simulink model "TEST_simulink"  (R2022b)
settings: Solver=VariableStepAuto  StartTime=0.0  StopTime=10.0  RelTol=1e-3
undefined symbols (not defined in the file): c0, c1, GFl_Final_vlaue, GFl_Initial_value, GFl_P_primary, GFl_Q_set, GFl_Sample_time, GFl_Step_time, GFm_Final_vlaue, GFm_Initial_value, GFm_P_primary, GFm_Q_set, GFm_Sample_time, GFm_Step_time, GFm_V_set_phph, GFmAIC_f_set, GFmAIC_Final_vlaue, GFmAIC_Initial_value, GFmAIC_P_primary, GFmAIC_P_set, GFmAIC_Q_set, GFmAIC_Sample_time, GFmAIC_Step_time, l0, l1, r0, r1, SG_f_set, SG_Final_vlaue, SG_Initial_value, SG_P_primary, SG_Q_set, SG_Sample_time, SG_Step_time, SG_V_set_phph, sigbuilder_block, V1_L1, V1_Ph_Ph, V1_R1, V2_L1, V2_Ph_Ph, V2_R1
libraries: Model_DG_Grid_Forming_Converter x30, Model_DG_Grid_Following_Converter x15, simulink x15, Model_DG_Synchronous_Generator x15, spsThreePhaseVIMeasurementLib x14, spsThreePhasePISectionLineLib x14, spsThreePhaseBreakerLib x6, spsThreePhaseFaultLib x3, spsThreePhaseParallelRLCLoadLib x2, spsThreePhaseTransformerTwoWindingsLib x2, spspowerguiLib x1
(part 4 of 6)

== system TEST_simulink/DER 2/Grid Forming Conventer ==
  Bus Selector : BusSelector  OutputSignals=controller.measurements.P_grid,controller.measurements.Q_grid,controller.inner_control.f,physical.V_dc,physical.V_grid_abc
  Constant : Constant  Value=GFm_P_primary
  Constant10 : Constant  Value=GFm_Q_set
  Constant4 : Constant  Value=GFmAIC_f_set
  Constant6 : Constant  Value=GFm_V_set_phph
  Grid_Forming_Converter1 : Model_DG_Grid_Forming_Converter/Grid_Forming_Converter  S_n=2e6  V_n_phph=690  f_n=50  send_messages=on  T_s_ctrl=1e-4  T_s_PWM_meas=1e-4  T_s_SPS=1e-4  datatype='double'  swModeling=Average Model  f_sw=5e3  L_filter_conv_pu=[ 0.001 0.05097 ]  C_filter_pu=[ 0.06875 0.04569 ]  L_filter_grid_pu=[ 0.01 0.04 ]  C_dc_pu=0.75  withTransformer=Grid coupling using transformer  V_n_grid_phph=20e3  RL_Trafo_Conv=[ 0.005 0.02 ]  RL_Trafo_Grid=[ 0.005 0.02 ]  Rm=500  Lm=500  meas_lowpass=on  meas_f_cutoff_lowpass=2500  meas_f_cutoff_posseq=20  prot_variant=tDMSquared warnings only  v_dc_max=1.2  v_ac_max=1.4  t_ac_max=0.1  v_ac_maxmax=1.25  t_ac_maxmax=0.1  v_ac_min=0.8  t_ac_min=3  v_ac_minmin=0.45  t_ac_minmin=0.3  f_ac_max=51.5  t_f_ac_max=0.1  f_ac_maxmax=52.5  t_f_ac_maxmax=10  f_ac_min=47.5  t_f_ac_min=0.1  i_ac_max=1.3  outerCtrlStrategy=Droop  OuterCtrl_droop_kP=0.05  OuterCtrl_droop_kQ=0.1  OuterCtrl_droop_TQ=0.2  OuterCtrl_ZDroop_kf=0.05  OuterCtrl_ZDroop_kV=0.1  OuterCtrl_ZDroop_kR=0  OuterCtrl_ZDroop_kX=1  OuterCtrl_ZDroop_TV=0.2  OuterCtrl_VSM_H=0.1  OuterCtrl_VSM_Kd=40  OuterCtrl_VSM_K=20  OuterCtrl_VSM_kQ=0.1  OuterCtrl_VSM_TQ=0.2  OuterCtrl_Dual_Kp=0.01  OuterCtrl_Dual_Kd=1e-4  OuterCtrl_Dual_kQ=0.1  OuterCtrl_Dual_TQ=0.2  OuterCtrl_Lvirt=0  InnerCtrl_K_p_V_cap_controller=0.8  InnerCtrl_K_i_V_cap_controller=0.5  InnerCtrl_K_p_I_conv_controller=3.3  InnerCtrl_K_i_I_conv_controller=16.5  InnerCtrl_v_conv_max=1.3  InnerCtrl_i_conv_max=1  InnerCtrl_Cff_V_cap_ctrl=disabled  InnerCtrl_Cff_I_conv_ctrl=disabled  InnerCtrl_K_ff_I_grid=enabled  InnerCtrl_K_ff_V_cap=enabled  InnerCtrl_i_lim_type=dq coordinate system  InnerCtrl_active_damping=enabled  InnerCtrl_AD_R_virt_pu=0.2
      settings: SourceProductName=tDMSquared
  Ground : Ground
  P_set_1 : Subsystem  Tag=STV Subsys  LoadFcn=sigbuilder_block('load');  StartFcn=sigbuilder_block('start');  StopFcn=sigbuilder_block('stop');  ClipboardFcn=sigbuilder_block('clipboard');  mask(Sigbuilder block){tuvar=[0:10]}
      mask help: Simulink:masks:SigbuilderBlock_MD
      mask init:
      | if ~strcmp(get_param(bdroot(gcbh),'SimulationStatus'),'stopped') tuvar = sigbuilder_block('maskInit'); end
      settings: CopyFcn=sigbuilder_block('copy');  DeleteFcn=sigbuilder_block('delete');  ModelCloseFcn=sigbuilder_block('modelClose');  PreSaveFcn=sigbuilder_block('preSave');  PauseFcn=sigbuilder_block('pause');  ContinueFcn=sigbuilder_block('continue');  NameChangeFcn=sigbuilder_block('namechange');  OpenFcn=sigbuilder_block('open',[-809.4 12.6 550.8 361.2 ]);  CloseFcn=sigbuilder_block('close');
      mask Display: plot(0, 0, 100, 100,[2, 2, 32, 32, 2], [68, 8, 8, 68, 68],[32, 2], [38, 38], [32, 19, 2],[53, 60, 44], [32, 17, 17, 2],[16, 16, 31, 31]);txt = getActiveGroup(gcbh);text(2, 100, txt,'verticalAlignment', 'top');
  Scope{,1..5} (6 alike) : Scope
  Step5 : Step  Time=GFm_Step_time  Before=GFm_Initial_value  After=GFm_Final_vlaue  SampleTime=GFm_Sample_time
  a : PMIOPort  Side=Right
  b : PMIOPort  Port=2  Side=Right
  c : PMIOPort  Port=3  Side=Right
  wires:
  [conv_1] -> Bus Selector/1
  Grid_Forming_Converter1/1 -> [conv_1]
  Bus Selector/4 -> Scope4/1  "<V_dc>"
  Bus Selector/1 -> Scope1/1  "<P_grid>"
  Bus Selector/3 -> Scope3/1  "<f>"
  Bus Selector/2 -> Scope2/1  "<Q_grid>"
  Bus Selector/5 -> Scope5/1  "<V_grid_abc>"
  P_set_1/1(P_set_1) -> Scope/1, Grid_Forming_Converter1/2
  Constant/1 -> Grid_Forming_Converter1/1
  Constant10/1 -> Grid_Forming_Converter1/3
  Constant4/1 -> Grid_Forming_Converter1/4
  Constant6/1 -> Grid_Forming_Converter1/5
  Ground/1 -> Grid_Forming_Converter1/6
  Step5/1 -> Grid_Forming_Converter1/7
  connections:
  c/RConn1 -- Grid_Forming_Converter1/RConn3
  b/RConn1 -- Grid_Forming_Converter1/RConn2
  a/RConn1 -- Grid_Forming_Converter1/RConn1

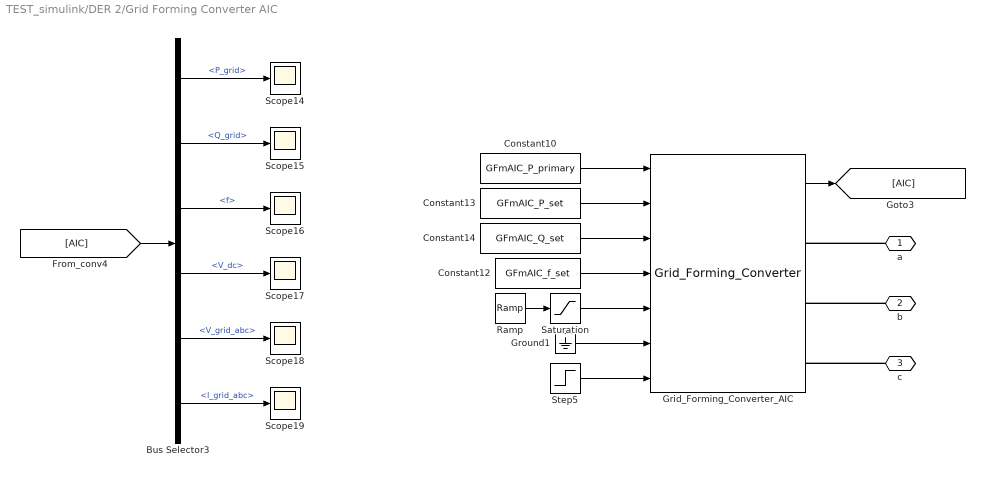
== system TEST_simulink/DER 2/Grid Forming Converter AIC ==
  Bus Selector3 : BusSelector  OutputSignals=controller.measurements.P_grid,controller.measurements.Q_grid,controller.inner_control.f,physical.V_dc,physical.V_grid_abc,physical.I_grid_abc
  Constant10 : Constant  Value=GFmAIC_P_primary
  Constant12 : Constant  Value=GFmAIC_f_set
  Constant13 : Constant  Value=GFmAIC_P_set
  Constant14 : Constant  Value=GFmAIC_Q_set
  Grid_Forming_Converter_AIC : Model_DG_Grid_Forming_Converter/Grid_Forming_Converter  S_n=100e3  V_n_phph=400  f_n=50  send_messages=on  T_s_ctrl=2e-4  T_s_PWM_meas=1e-5  T_s_SPS=1e-5  datatype='double'  swModeling=Average Model  f_sw=2.5e3  L_filter_conv_pu=[ 0.001 0.0177 ]  C_filter_pu=[ 0.000104 0.213 ]  L_filter_grid_pu=[ 0.001 0.00432 ]  C_dc_pu=0.75  withTransformer=Direct grid coupling of converter  V_n_grid_phph=400  RL_Trafo_Conv=[ 0.005 0.02 ]  RL_Trafo_Grid=[ 0.005 0.02 ]  Rm=500  Lm=500  meas_lowpass=on  meas_f_cutoff_lowpass=2500  meas_f_cutoff_posseq=20  prot_variant=tDMSquared warnings only  v_dc_max=1.2  v_ac_max=1.4  t_ac_max=0.1  v_ac_maxmax=1.25  t_ac_maxmax=0.1  v_ac_min=0.8  t_ac_min=3  v_ac_minmin=0.45  t_ac_minmin=0.3  f_ac_max=51.5  t_f_ac_max=0.1  f_ac_maxmax=52.5  t_f_ac_maxmax=10  f_ac_min=47.5  t_f_ac_min=0.1  i_ac_max=1.3  outerCtrlStrategy=Droop  OuterCtrl_droop_kP=0.05  OuterCtrl_droop_kQ=0.1  OuterCtrl_droop_TQ=0.2  OuterCtrl_ZDroop_kf=0.05  OuterCtrl_ZDroop_kV=0.1  OuterCtrl_ZDroop_kR=0  OuterCtrl_ZDroop_kX=1  OuterCtrl_ZDroop_TV=0.2  OuterCtrl_VSM_H=0.1  OuterCtrl_VSM_Kd=40  OuterCtrl_VSM_K=20  OuterCtrl_VSM_kQ=0.1  OuterCtrl_VSM_TQ=0.2  OuterCtrl_Dual_Kp=0.01  OuterCtrl_Dual_Kd=1e-4  OuterCtrl_Dual_kQ=0.1  OuterCtrl_Dual_TQ=0.2  OuterCtrl_Lvirt=0  InnerCtrl_K_p_V_cap_controller=0.17  InnerCtrl_K_i_V_cap_controller=4.24  InnerCtrl_K_p_I_conv_controller=0.5  InnerCtrl_K_i_I_conv_controller=2.5  InnerCtrl_v_conv_max=1.3  InnerCtrl_i_conv_max=1.32  InnerCtrl_Cff_V_cap_ctrl=disabled  InnerCtrl_Cff_I_conv_ctrl=disabled  InnerCtrl_K_ff_I_grid=enabled  InnerCtrl_K_ff_V_cap=enabled  InnerCtrl_i_lim_type=abc coordinate system  InnerCtrl_active_damping=enabled  InnerCtrl_AD_R_virt_pu=0.1
      settings: SourceProductName=tDMSquared
  Ground1 : Ground
  Ramp : simulink/Sources/Ramp  slope=400  start=0  InitialOutput=0
  Saturation : Saturate  UpperLimit=400
  Scope{14..19} (6 alike) : Scope
  Step5 : Step  Time=GFmAIC_Step_time  Before=GFmAIC_Initial_value  After=GFmAIC_Final_vlaue  SampleTime=GFmAIC_Sample_time
  a : PMIOPort  Side=Right
  b : PMIOPort  Port=2  Side=Right
  c : PMIOPort  Port=3  Side=Right
  wires:
  Bus Selector3/1 -> Scope14/1  "<P_grid>"
  Constant13/1 -> Grid_Forming_Converter_AIC/2
  Saturation/1 -> Grid_Forming_Converter_AIC/5
  Constant10/1 -> Grid_Forming_Converter_AIC/1
  Ramp/1 -> Saturation/1
  Constant12/1 -> Grid_Forming_Converter_AIC/4
  Ground1/1 -> Grid_Forming_Converter_AIC/6
  Bus Selector3/4 -> Scope17/1  "<V_dc>"
  Bus Selector3/3 -> Scope16/1  "<f>"
  Grid_Forming_Converter_AIC/1 -> [AIC]
  Constant14/1 -> Grid_Forming_Converter_AIC/3
  Bus Selector3/5 -> Scope18/1  "<V_grid_abc>"
  [AIC] -> Bus Selector3/1
  Bus Selector3/6 -> Scope19/1  "<I_grid_abc>"
  Bus Selector3/2 -> Scope15/1  "<Q_grid>"
  Step5/1 -> Grid_Forming_Converter_AIC/7
  connections:
  b/RConn1 -- Grid_Forming_Converter_AIC/RConn2
  a/RConn1 -- Grid_Forming_Converter_AIC/RConn1
  c/RConn1 -- Grid_Forming_Converter_AIC/RConn3

== system TEST_simulink/DER 2/SG ==
  Bus Selector2 : BusSelector  OutputSignals=electrical_SI.P_grid_SI,electrical_SI.Q_grid_SI,SG_SI.Frequency (Hz),electrical_SI.V_grid_SI
  Constant1 : Constant  Value=SG_P_primary
  Constant3 : Constant  Value=SG_f_set
  Constant5 : Constant  Value=SG_Q_set
  Constant7 : Constant  Value=SG_V_set_phph
  P_set_2 : Subsystem  Tag=STV Subsys  LoadFcn=sigbuilder_block('load');  StartFcn=sigbuilder_block('start');  StopFcn=sigbuilder_block('stop');  ClipboardFcn=sigbuilder_block('clipboard');  mask(Sigbuilder block){tuvar=[0:10]}
      mask help: Simulink:masks:SigbuilderBlock_MD
      mask init:
      | if ~strcmp(get_param(bdroot(gcbh),'SimulationStatus'),'stopped') tuvar = sigbuilder_block('maskInit'); end
      settings: CopyFcn=sigbuilder_block('copy');  DeleteFcn=sigbuilder_block('delete');  ModelCloseFcn=sigbuilder_block('modelClose');  PreSaveFcn=sigbuilder_block('preSave');  PauseFcn=sigbuilder_block('pause');  ContinueFcn=sigbuilder_block('continue');  NameChangeFcn=sigbuilder_block('namechange');  OpenFcn=sigbuilder_block('open',[665.4 126 550.8 400.2 ]);  CloseFcn=sigbuilder_block('close');
      mask Display: plot(0, 0, 100, 100,[2, 2, 32, 32, 2], [68, 8, 8, 68, 68],[32, 2], [38, 38], [32, 19, 2],[53, 60, 44], [32, 17, 17, 2],[16, 16, 31, 31]);txt = getActiveGroup(gcbh);text(2, 100, txt,'verticalAlignment', 'top');
  Scope{7..9,11} (4 alike) : Scope
  Step2 : Step  Time=SG_Step_time  Before=SG_Initial_value  After=SG_Final_vlaue  SampleTime=SG_Sample_time
  Synchronous_Generator : Model_DG_Synchronous_Generator/Synchronous_Generator  S_n=3.2e6  P_binst=2.0e6  V_n_phph=400  V_n_grid_phph=20e3  f_n=50  T_s_ctrl=1e-4  T_s_meas=1e-4  datatype='double'  SG_Reactances=[ 3.19 0.33 0.159 1.79 0.155 0.05 ]  SG_TimeConstants=[ 0.5 0.025 0.025 ]  SG_StatorResistance=0.00074  SG_mech=[ 0.366 0.01 2 ]  gov_type=IEEEG1 simplified  K_IEEEG1simp=10  T_IEEEG1simp=[ 0.2 0 0.1 0 ]  dP_maxmin_IEEEG1simp=[ 2 -2 ]  exciterModel=AC1A  QCtrl=Constant Voltage (no Q-Control)  K_p_QCtrl=0.5  K_i_QCtrl=0.4  uq0ref=1.0  qmax=0.33  umax=1.04  deadband=0  p_pu=[0.1, 0.5, 0.6, 0.9, 1.0]  q_pu=[0.0, 0.0, -0.05, -0.33, -0.33]  p1=[0.94, 0.33]  p2=[0.96, 0]  p3=[1.04, 0]  p4=[1.06, -0.33]  cosphi_ref=1  ind_cap_Q=Inductive behavior (capacitive Q infeed)  use_transformer=Grid coupling with transformer  RL_Trafo_GenSide=[ 0.002 0.08 ]  RL_Trafo_GridSide=[ 0.002 0.08 ]  Trafo_RmLm=[ 500 500 ]
      link override SG_Control/Exciter: LabelModeActiveChoice=AC1A
      link override SG_Control/Reactive_Power_Controller: LabelModeActiveChoice=const_V
      settings: SourceProductName=tDMSquared
  a : PMIOPort  Side=Right
  b : PMIOPort  Port=2  Side=Right
  c : PMIOPort  Port=3  Side=Right
  wires:
  Synchronous_Generator/1 -> [sg]
  [sg] -> Bus Selector2/1
  Bus Selector2/3 -> Scope9/1  "<Frequency (Hz)>"
  Bus Selector2/1 -> Scope7/1  "<P_grid_SI>"
  Bus Selector2/2 -> Scope8/1  "<Q_grid_SI>"
  Bus Selector2/4 -> Scope11/1  "<V_grid_SI>"
  Constant5/1 -> Synchronous_Generator/3
  Constant1/1 -> Synchronous_Generator/1
  P_set_2/1(P_set_2) -> Synchronous_Generator/2
  Constant3/1 -> Synchronous_Generator/4
  Constant7/1 -> Synchronous_Generator/5
  Step2/1 -> Synchronous_Generator/6
  connections:
  b/RConn1 -- Synchronous_Generator/RConn2
  c/RConn1 -- Synchronous_Generator/RConn3
  a/RConn1 -- Synchronous_Generator/RConn1

== system TEST_simulink/DER 3/Grid Following Conventer ==
  Bus Selector1 : BusSelector  OutputSignals=controller.measurements.P_grid,controller.measurements.Q_grid,controller.PLL.f_PLL,physical.V_grid_abc
  Constant8 : Constant  Value=GFl_P_primary
  Constant9 : Constant  Value=GFl_Q_set
  Gain : Gain  Gain=50
  Grid-Following Converter (3-phase)1 : Model_DG_Grid_Following_Converter/Grid-Following Converter (3-phase)  S_n=2e6  P_binst=1.5e6  V_n_phph=690  f_n=50  send_messages=on  T_s_ctrl=1e-3  T_s_PWM_meas=1e-4  T_s_SPS=1e-4  datatype='double'  swModeling=Average Model  f_sw=5e3  L_filter_conv_pu=[ 0.005 0.23 ]  C_filter_pu=[ 0.005 0.01 ]  L_filter_grid_pu=[ 0.01 0.04 ]  withTransformer=Grid coupling using transformer  V_n_grid_phph=20e3  RL_Trafo_Conv=[ 0.005 0.02 ]  RL_Trafo_Grid=[ 0.005 0.02 ]  Rm=500  Lm=500  meas_LPF=on  meas_LPF_f_cutoff=2500  prot_variant=tDMSquared warnings only  prot_v_ac_max=1.4  prot_t_ac_max=0.1  prot_v_ac_maxmax=1.25  prot_t_ac_maxmax=0.1  prot_v_ac_min=0.8  prot_t_ac_min=3  prot_v_ac_minmin=0.45  prot_t_ac_minmin=0.3  prot_f_ac_max=51.5  prot_t_f_ac_max=0.1  prot_f_ac_maxmax=52.5  prot_t_f_ac_maxmax=10  prot_f_ac_min=47.5  prot_t_f_ac_min=0.1  prot_i_ac_max=1.3  unitCtrlMode=VDE 4110  VDE4110_Pf_DBlow=49.8  VDE4110_Pf_DBhigh=50.2  VDE4110_Pf_droop=5  VDE4110_Pf_dPdt_max=1  VDE4110_Pf_T_LPF=33e-3  VDE4110_Pf_isStorage=on  VDE4110_Q_Mode=(c) Constant Q with Q(V)-limitation  VDE4110_Q_T_PT1=3.33  VDE4110_uq0ref=1  VDE4110_qmax=0.33  VDE4110_umax=1.04  VDE4110_deadband=0  VDE4110_p_pu=[0.1, 0.5, 0.6, 0.9, 1.0]  VDE4110_q_pu=[0.0, 0.0, -0.05, -0.33, -0.33]  VDE4110_p1=[0.94, 0.33]  VDE4110_p2=[0.96, 0]  VDE4110_p3=[1.04, 0]  VDE4110_p4=[1.06, -0.33]  VDE4110_cosphi_ref=1  VDE4110_Q_direction=Inductive Q injection  InnerCtrl_PQ_Ctrl_Mode=Closed loop  InnerCtrl_Kp_PQ=1  InnerCtrl_Ki_PQ=5  InnerCtrl_Kp=0.3  InnerCtrl_Ki=2  InnerCtrl_v_conv_max=1.25  InnerCtrl_i_conv_max=1.1  InnerCtrl_AD_activated=on  InnerCtrl_AD_Rvirt=0.1
      settings: SourceProductName=tDMSquared
  P_set_3 : Subsystem  Tag=STV Subsys  LoadFcn=sigbuilder_block('load');  StartFcn=sigbuilder_block('start');  StopFcn=sigbuilder_block('stop');  ClipboardFcn=sigbuilder_block('clipboard');  mask(Sigbuilder block){tuvar=[0:10]}
      mask help: Simulink:masks:SigbuilderBlock_MD
      mask init:
      | if ~strcmp(get_param(bdroot(gcbh),'SimulationStatus'),'stopped') tuvar = sigbuilder_block('maskInit'); end
      settings: CopyFcn=sigbuilder_block('copy');  DeleteFcn=sigbuilder_block('delete');  ModelCloseFcn=sigbuilder_block('modelClose');  PreSaveFcn=sigbuilder_block('preSave');  PauseFcn=sigbuilder_block('pause');  ContinueFcn=sigbuilder_block('continue');  NameChangeFcn=sigbuilder_block('namechange');  OpenFcn=sigbuilder_block('open',[-809.4 12.6 550.8 361.2 ]);  CloseFcn=sigbuilder_block('close');
      mask Display: plot(0, 0, 100, 100,[2, 2, 32, 32, 2], [68, 8, 8, 68, 68],[32, 2], [38, 38], [32, 19, 2],[53, 60, 44], [32, 17, 17, 2],[16, 16, 31, 31]);txt = getActiveGroup(gcbh);text(2, 100, txt,'verticalAlignment', 'top');
  Scope{6,10,12..13} (4 alike) : Scope
  Step5 : Step  Time=GFl_Step_time  Before=GFl_Initial_value  After=GFl_Final_vlaue  SampleTime=GFl_Sample_time
  a : PMIOPort  Side=Right
  b : PMIOPort  Port=2  Side=Right
  c : PMIOPort  Port=3  Side=Right
  wires:
  Grid-Following Converter (3-phase)1/1 -> [conv_1]
  Gain/1 -> Scope12/1
  [conv_1] -> Bus Selector1/1
  Bus Selector1/4 -> Scope13/1  "<V_grid_abc>"
  Bus Selector1/1 -> Scope6/1  "<P_grid>"
  Bus Selector1/2 -> Scope10/1  "<Q_grid>"
  Bus Selector1/3 -> Gain/1  "<f_PLL>"
  Step5/1 -> Grid-Following Converter (3-phase)1/4
  Constant8/1 -> Grid-Following Converter (3-phase)1/1
  P_set_3/1(P_set_1) -> Grid-Following Converter (3-phase)1/2
  Constant9/1 -> Grid-Following Converter (3-phase)1/3
  connections:
  Grid-Following Converter (3-phase)1/RConn3 -- c/RConn1
  Grid-Following Converter (3-phase)1/RConn1 -- a/RConn1
  Grid-Following Converter (3-phase)1/RConn2 -- b/RConn1

== system TEST_simulink/DER 3/Grid Forming Conventer ==
  Bus Selector : BusSelector  OutputSignals=controller.measurements.P_grid,controller.measurements.Q_grid,controller.inner_control.f,physical.V_dc,physical.V_grid_abc
  Constant11 : Constant  Value=GFm_P_primary
  Constant15 : Constant  Value=GFm_Q_set
  Constant16 : Constant  Value=GFmAIC_f_set
  Constant17 : Constant  Value=GFm_V_set_phph
  Grid_Forming_Converter1 : Model_DG_Grid_Forming_Converter/Grid_Forming_Converter  S_n=2e6  V_n_phph=690  f_n=50  send_messages=on  T_s_ctrl=1e-4  T_s_PWM_meas=1e-4  T_s_SPS=1e-4  datatype='double'  swModeling=Average Model  f_sw=5e3  L_filter_conv_pu=[ 0.001 0.05097 ]  C_filter_pu=[ 0.06875 0.04569 ]  L_filter_grid_pu=[ 0.01 0.04 ]  C_dc_pu=0.75  withTransformer=Grid coupling using transformer  V_n_grid_phph=20e3  RL_Trafo_Conv=[ 0.005 0.02 ]  RL_Trafo_Grid=[ 0.005 0.02 ]  Rm=500  Lm=500  meas_lowpass=on  meas_f_cutoff_lowpass=2500  meas_f_cutoff_posseq=20  prot_variant=tDMSquared warnings only  v_dc_max=1.2  v_ac_max=1.4  t_ac_max=0.1  v_ac_maxmax=1.25  t_ac_maxmax=0.1  v_ac_min=0.8  t_ac_min=3  v_ac_minmin=0.45  t_ac_minmin=0.3  f_ac_max=51.5  t_f_ac_max=0.1  f_ac_maxmax=52.5  t_f_ac_maxmax=10  f_ac_min=47.5  t_f_ac_min=0.1  i_ac_max=1.3  outerCtrlStrategy=Droop  OuterCtrl_droop_kP=0.05  OuterCtrl_droop_kQ=0.1  OuterCtrl_droop_TQ=0.2  OuterCtrl_ZDroop_kf=0.05  OuterCtrl_ZDroop_kV=0.1  OuterCtrl_ZDroop_kR=0  OuterCtrl_ZDroop_kX=1  OuterCtrl_ZDroop_TV=0.2  OuterCtrl_VSM_H=0.1  OuterCtrl_VSM_Kd=40  OuterCtrl_VSM_K=20  OuterCtrl_VSM_kQ=0.1  OuterCtrl_VSM_TQ=0.2  OuterCtrl_Dual_Kp=0.01  OuterCtrl_Dual_Kd=1e-4  OuterCtrl_Dual_kQ=0.1  OuterCtrl_Dual_TQ=0.2  OuterCtrl_Lvirt=0  InnerCtrl_K_p_V_cap_controller=0.8  InnerCtrl_K_i_V_cap_controller=0.5  InnerCtrl_K_p_I_conv_controller=3.3  InnerCtrl_K_i_I_conv_controller=16.5  InnerCtrl_v_conv_max=1.3  InnerCtrl_i_conv_max=1  InnerCtrl_Cff_V_cap_ctrl=disabled  InnerCtrl_Cff_I_conv_ctrl=disabled  InnerCtrl_K_ff_I_grid=enabled  InnerCtrl_K_ff_V_cap=enabled  InnerCtrl_i_lim_type=dq coordinate system  InnerCtrl_active_damping=enabled  InnerCtrl_AD_R_virt_pu=0.2
      settings: SourceProductName=tDMSquared
  Ground2 : Ground
  P_set_4 : Subsystem  Tag=STV Subsys  LoadFcn=sigbuilder_block('load');  StartFcn=sigbuilder_block('start');  StopFcn=sigbuilder_block('stop');  ClipboardFcn=sigbuilder_block('clipboard');  mask(Sigbuilder block){tuvar=[0:10]}
      mask help: Simulink:masks:SigbuilderBlock_MD
      mask init:
      | if ~strcmp(get_param(bdroot(gcbh),'SimulationStatus'),'stopped') tuvar = sigbuilder_block('maskInit'); end
      settings: CopyFcn=sigbuilder_block('copy');  DeleteFcn=sigbuilder_block('delete');  ModelCloseFcn=sigbuilder_block('modelClose');  PreSaveFcn=sigbuilder_block('preSave');  PauseFcn=sigbuilder_block('pause');  ContinueFcn=sigbuilder_block('continue');  NameChangeFcn=sigbuilder_block('namechange');  OpenFcn=sigbuilder_block('open',[-809.4 12.6 550.8 361.2 ]);  CloseFcn=sigbuilder_block('close');
      mask Display: plot(0, 0, 100, 100,[2, 2, 32, 32, 2], [68, 8, 8, 68, 68],[32, 2], [38, 38], [32, 19, 2],[53, 60, 44], [32, 17, 17, 2],[16, 16, 31, 31]);txt = getActiveGroup(gcbh);text(2, 100, txt,'verticalAlignment', 'top');
  Scope{1..5} (5 alike) : Scope
  Step4 : Step  Time=GFm_Step_time  Before=GFm_Initial_value  After=GFm_Final_vlaue  SampleTime=GFm_Sample_time
  a : PMIOPort  Side=Right
  b : PMIOPort  Port=2  Side=Right
  c : PMIOPort  Port=3  Side=Right
  wires:
  Bus Selector/5 -> Scope5/1  "<V_grid_abc>"
  Bus Selector/2 -> Scope2/1  "<Q_grid>"
  Bus Selector/3 -> Scope3/1  "<f>"
  Bus Selector/1 -> Scope1/1  "<P_grid>"
  Bus Selector/4 -> Scope4/1  "<V_dc>"
  Grid_Forming_Converter1/1 -> [conv_1]
  [conv_1] -> Bus Selector/1
  Constant15/1 -> Grid_Forming_Converter1/3
  Ground2/1 -> Grid_Forming_Converter1/6
  Step4/1 -> Grid_Forming_Converter1/7
  Constant17/1 -> Grid_Forming_Converter1/5
  P_set_4/1(P_set_1) -> Grid_Forming_Converter1/2
  Constant11/1 -> Grid_Forming_Converter1/1
  Constant16/1 -> Grid_Forming_Converter1/4
  connections:
  Grid_Forming_Converter1/RConn3 -- c/RConn1
  Grid_Forming_Converter1/RConn1 -- a/RConn1
  Grid_Forming_Converter1/RConn2 -- b/RConn1

== system TEST_simulink/DER 3/Grid Forming Converter AIC ==
  Bus Selector3 : BusSelector  OutputSignals=controller.measurements.P_grid,controller.measurements.Q_grid,controller.inner_control.f,physical.V_dc,physical.V_grid_abc,physical.I_grid_abc
  Constant11 : Constant  Value=GFm_P_primary
  Constant15 : Constant  Value=GFm_Q_set
  Constant16 : Constant  Value=GFmAIC_f_set
  Constant17 : Constant  Value=GFm_V_set_phph
  Grid_Forming_Converter_AIC : Model_DG_Grid_Forming_Converter/Grid_Forming_Converter  S_n=100e3  V_n_phph=400  f_n=50  send_messages=on  T_s_ctrl=2e-4  T_s_PWM_meas=1e-5  T_s_SPS=1e-5  datatype='double'  swModeling=Average Model  f_sw=2.5e3  L_filter_conv_pu=[ 0.001 0.0177 ]  C_filter_pu=[ 0.000104 0.213 ]  L_filter_grid_pu=[ 0.001 0.00432 ]  C_dc_pu=0.75  withTransformer=Direct grid coupling of converter  V_n_grid_phph=400  RL_Trafo_Conv=[ 0.005 0.02 ]  RL_Trafo_Grid=[ 0.005 0.02 ]  Rm=500  Lm=500  meas_lowpass=on  meas_f_cutoff_lowpass=2500  meas_f_cutoff_posseq=20  prot_variant=tDMSquared warnings only  v_dc_max=1.2  v_ac_max=1.4  t_ac_max=0.1  v_ac_maxmax=1.25  t_ac_maxmax=0.1  v_ac_min=0.8  t_ac_min=3  v_ac_minmin=0.45  t_ac_minmin=0.3  f_ac_max=51.5  t_f_ac_max=0.1  f_ac_maxmax=52.5  t_f_ac_maxmax=10  f_ac_min=47.5  t_f_ac_min=0.1  i_ac_max=1.3  outerCtrlStrategy=Droop  OuterCtrl_droop_kP=0.05  OuterCtrl_droop_kQ=0.1  OuterCtrl_droop_TQ=0.2  OuterCtrl_ZDroop_kf=0.05  OuterCtrl_ZDroop_kV=0.1  OuterCtrl_ZDroop_kR=0  OuterCtrl_ZDroop_kX=1  OuterCtrl_ZDroop_TV=0.2  OuterCtrl_VSM_H=0.1  OuterCtrl_VSM_Kd=40  OuterCtrl_VSM_K=20  OuterCtrl_VSM_kQ=0.1  OuterCtrl_VSM_TQ=0.2  OuterCtrl_Dual_Kp=0.01  OuterCtrl_Dual_Kd=1e-4  OuterCtrl_Dual_kQ=0.1  OuterCtrl_Dual_TQ=0.2  OuterCtrl_Lvirt=0  InnerCtrl_K_p_V_cap_controller=0.17  InnerCtrl_K_i_V_cap_controller=4.24  InnerCtrl_K_p_I_conv_controller=0.5  InnerCtrl_K_i_I_conv_controller=2.5  InnerCtrl_v_conv_max=1.3  InnerCtrl_i_conv_max=1.32  InnerCtrl_Cff_V_cap_ctrl=disabled  InnerCtrl_Cff_I_conv_ctrl=disabled  InnerCtrl_K_ff_I_grid=enabled  InnerCtrl_K_ff_V_cap=enabled  InnerCtrl_i_lim_type=abc coordinate system  InnerCtrl_active_damping=enabled  InnerCtrl_AD_R_virt_pu=0.1
      settings: SourceProductName=tDMSquared
  Ground2 : Ground
  P_set_4 : Subsystem  Tag=STV Subsys  LoadFcn=sigbuilder_block('load');  StartFcn=sigbuilder_block('start');  StopFcn=sigbuilder_block('stop');  ClipboardFcn=sigbuilder_block('clipboard');  mask(Sigbuilder block){tuvar=[0:10]}
      mask help: Simulink:masks:SigbuilderBlock_MD
      mask init:
      | if ~strcmp(get_param(bdroot(gcbh),'SimulationStatus'),'stopped') tuvar = sigbuilder_block('maskInit'); end
      settings: CopyFcn=sigbuilder_block('copy');  DeleteFcn=sigbuilder_block('delete');  ModelCloseFcn=sigbuilder_block('modelClose');  PreSaveFcn=sigbuilder_block('preSave');  PauseFcn=sigbuilder_block('pause');  ContinueFcn=sigbuilder_block('continue');  NameChangeFcn=sigbuilder_block('namechange');  OpenFcn=sigbuilder_block('open',[-809.4 12.6 550.8 361.2 ]);  CloseFcn=sigbuilder_block('close');
      mask Display: plot(0, 0, 100, 100,[2, 2, 32, 32, 2], [68, 8, 8, 68, 68],[32, 2], [38, 38], [32, 19, 2],[53, 60, 44], [32, 17, 17, 2],[16, 16, 31, 31]);txt = getActiveGroup(gcbh);text(2, 100, txt,'verticalAlignment', 'top');
  Scope{14..19} (6 alike) : Scope
  Step4 : Step  Time=GFm_Step_time  Before=GFm_Initial_value  After=GFm_Final_vlaue  SampleTime=GFm_Sample_time
  a : PMIOPort  Side=Right
  b : PMIOPort  Port=2  Side=Right
  c : PMIOPort  Port=3  Side=Right
  wires:
  Bus Selector3/2 -> Scope15/1  "<Q_grid>"
  Bus Selector3/6 -> Scope19/1  "<I_grid_abc>"
  [AIC] -> Bus Selector3/1
  Bus Selector3/5 -> Scope18/1  "<V_grid_abc>"
  Grid_Forming_Converter_AIC/1 -> [AIC]
  Bus Selector3/3 -> Scope16/1  "<f>"
  Bus Selector3/4 -> Scope17/1  "<V_dc>"
  Bus Selector3/1 -> Scope14/1  "<P_grid>"
  Constant15/1 -> Grid_Forming_Converter_AIC/3
  Ground2/1 -> Grid_Forming_Converter_AIC/6
  Step4/1 -> Grid_Forming_Converter_AIC/7
  Constant17/1 -> Grid_Forming_Converter_AIC/5
  P_set_4/1(P_set_1) -> Grid_Forming_Converter_AIC/2
  Constant11/1 -> Grid_Forming_Converter_AIC/1
  Constant16/1 -> Grid_Forming_Converter_AIC/4
  connections:
  Grid_Forming_Converter_AIC/RConn3 -- c/RConn1
  Grid_Forming_Converter_AIC/RConn1 -- a/RConn1
  Grid_Forming_Converter_AIC/RConn2 -- b/RConn1

== system TEST_simulink/DER 3/SG ==
  Bus Selector2 : BusSelector  OutputSignals=electrical_SI.P_grid_SI,electrical_SI.Q_grid_SI,SG_SI.Frequency (Hz),electrical_SI.V_grid_SI
  Constant1 : Constant  Value=SG_P_primary
  Constant3 : Constant  Value=SG_f_set
  Constant5 : Constant  Value=SG_Q_set
  Constant7 : Constant  Value=SG_V_set_phph
  P_set_2 : Subsystem  Tag=STV Subsys  LoadFcn=sigbuilder_block('load');  StartFcn=sigbuilder_block('start');  StopFcn=sigbuilder_block('stop');  ClipboardFcn=sigbuilder_block('clipboard');  mask(Sigbuilder block){tuvar=[0:10]}
      mask help: Simulink:masks:SigbuilderBlock_MD
      mask init:
      | if ~strcmp(get_param(bdroot(gcbh),'SimulationStatus'),'stopped') tuvar = sigbuilder_block('maskInit'); end
      settings: CopyFcn=sigbuilder_block('copy');  DeleteFcn=sigbuilder_block('delete');  ModelCloseFcn=sigbuilder_block('modelClose');  PreSaveFcn=sigbuilder_block('preSave');  PauseFcn=sigbuilder_block('pause');  ContinueFcn=sigbuilder_block('continue');  NameChangeFcn=sigbuilder_block('namechange');  OpenFcn=sigbuilder_block('open',[665.4 126 550.8 400.2 ]);  CloseFcn=sigbuilder_block('close');
      mask Display: plot(0, 0, 100, 100,[2, 2, 32, 32, 2], [68, 8, 8, 68, 68],[32, 2], [38, 38], [32, 19, 2],[53, 60, 44], [32, 17, 17, 2],[16, 16, 31, 31]);txt = getActiveGroup(gcbh);text(2, 100, txt,'verticalAlignment', 'top');
  Scope{7..9,11} (4 alike) : Scope
  Step2 : Step  Time=SG_Step_time  Before=SG_Initial_value  After=SG_Final_vlaue  SampleTime=SG_Sample_time
  Synchronous_Generator : Model_DG_Synchronous_Generator/Synchronous_Generator  S_n=3.2e6  P_binst=2.0e6  V_n_phph=400  V_n_grid_phph=20e3  f_n=50  T_s_ctrl=1e-4  T_s_meas=1e-4  datatype='double'  SG_Reactances=[ 3.19 0.33 0.159 1.79 0.155 0.05 ]  SG_TimeConstants=[ 0.5 0.025 0.025 ]  SG_StatorResistance=0.00074  SG_mech=[ 0.366 0.01 2 ]  gov_type=IEEEG1 simplified  K_IEEEG1simp=10  T_IEEEG1simp=[ 0.2 0 0.1 0 ]  dP_maxmin_IEEEG1simp=[ 2 -2 ]  exciterModel=AC1A  QCtrl=Constant Voltage (no Q-Control)  K_p_QCtrl=0.5  K_i_QCtrl=0.4  uq0ref=1.0  qmax=0.33  umax=1.04  deadband=0  p_pu=[0.1, 0.5, 0.6, 0.9, 1.0]  q_pu=[0.0, 0.0, -0.05, -0.33, -0.33]  p1=[0.94, 0.33]  p2=[0.96, 0]  p3=[1.04, 0]  p4=[1.06, -0.33]  cosphi_ref=1  ind_cap_Q=Inductive behavior (capacitive Q infeed)  use_transformer=Grid coupling with transformer  RL_Trafo_GenSide=[ 0.002 0.08 ]  RL_Trafo_GridSide=[ 0.002 0.08 ]  Trafo_RmLm=[ 500 500 ]
      link override SG_Control/Exciter: LabelModeActiveChoice=AC1A
      link override SG_Control/Reactive_Power_Controller: LabelModeActiveChoice=const_V
      settings: SourceProductName=tDMSquared
  a : PMIOPort  Side=Right
  b : PMIOPort  Port=2  Side=Right
  c : PMIOPort  Port=3  Side=Right
  wires:
  Bus Selector2/4 -> Scope11/1  "<V_grid_SI>"
  Bus Selector2/2 -> Scope8/1  "<Q_grid_SI>"
  Bus Selector2/1 -> Scope7/1  "<P_grid_SI>"
  Bus Selector2/3 -> Scope9/1  "<Frequency (Hz)>"
  [sg] -> Bus Selector2/1
  Synchronous_Generator/1 -> [sg]
  Constant7/1 -> Synchronous_Generator/5
  Constant3/1 -> Synchronous_Generator/4
  Constant1/1 -> Synchronous_Generator/1
  P_set_2/1(P_set_2) -> Synchronous_Generator/2
  Step2/1 -> Synchronous_Generator/6
  Constant5/1 -> Synchronous_Generator/3
  connections:
  a/RConn1 -- Synchronous_Generator/RConn1
  c/RConn1 -- Synchronous_Generator/RConn3
  b/RConn1 -- Synchronous_Generator/RConn2

== system TEST_simulink/DER 4/Grid Following Conventer ==
  Bus Selector1 : BusSelector  OutputSignals=controller.measurements.P_grid,controller.measurements.Q_grid,controller.PLL.f_PLL,physical.V_grid_abc
  Constant8 : Constant  Value=GFl_P_primary
  Constant9 : Constant  Value=GFl_Q_set
  Gain : Gain  Gain=50
  Grid-Following Converter (3-phase)1 : Model_DG_Grid_Following_Converter/Grid-Following Converter (3-phase)  S_n=2e6  P_binst=1.5e6  V_n_phph=690  f_n=50  send_messages=on  T_s_ctrl=1e-3  T_s_PWM_meas=1e-4  T_s_SPS=1e-4  datatype='double'  swModeling=Average Model  f_sw=5e3  L_filter_conv_pu=[ 0.005 0.23 ]  C_filter_pu=[ 0.005 0.01 ]  L_filter_grid_pu=[ 0.01 0.04 ]  withTransformer=Grid coupling using transformer  V_n_grid_phph=20e3  RL_Trafo_Conv=[ 0.005 0.02 ]  RL_Trafo_Grid=[ 0.005 0.02 ]  Rm=500  Lm=500  meas_LPF=on  meas_LPF_f_cutoff=2500  prot_variant=tDMSquared warnings only  prot_v_ac_max=1.4  prot_t_ac_max=0.1  prot_v_ac_maxmax=1.25  prot_t_ac_maxmax=0.1  prot_v_ac_min=0.8  prot_t_ac_min=3  prot_v_ac_minmin=0.45  prot_t_ac_minmin=0.3  prot_f_ac_max=51.5  prot_t_f_ac_max=0.1  prot_f_ac_maxmax=52.5  prot_t_f_ac_maxmax=10  prot_f_ac_min=47.5  prot_t_f_ac_min=0.1  prot_i_ac_max=1.3  unitCtrlMode=VDE 4110  VDE4110_Pf_DBlow=49.8  VDE4110_Pf_DBhigh=50.2  VDE4110_Pf_droop=5  VDE4110_Pf_dPdt_max=1  VDE4110_Pf_T_LPF=33e-3  VDE4110_Pf_isStorage=on  VDE4110_Q_Mode=(c) Constant Q with Q(V)-limitation  VDE4110_Q_T_PT1=3.33  VDE4110_uq0ref=1  VDE4110_qmax=0.33  VDE4110_umax=1.04  VDE4110_deadband=0  VDE4110_p_pu=[0.1, 0.5, 0.6, 0.9, 1.0]  VDE4110_q_pu=[0.0, 0.0, -0.05, -0.33, -0.33]  VDE4110_p1=[0.94, 0.33]  VDE4110_p2=[0.96, 0]  VDE4110_p3=[1.04, 0]  VDE4110_p4=[1.06, -0.33]  VDE4110_cosphi_ref=1  VDE4110_Q_direction=Inductive Q injection  InnerCtrl_PQ_Ctrl_Mode=Closed loop  InnerCtrl_Kp_PQ=1  InnerCtrl_Ki_PQ=5  InnerCtrl_Kp=0.3  InnerCtrl_Ki=2  InnerCtrl_v_conv_max=1.25  InnerCtrl_i_conv_max=1.1  InnerCtrl_AD_activated=on  InnerCtrl_AD_Rvirt=0.1
      settings: SourceProductName=tDMSquared
  P_set_3 : Subsystem  Tag=STV Subsys  LoadFcn=sigbuilder_block('load');  StartFcn=sigbuilder_block('start');  StopFcn=sigbuilder_block('stop');  ClipboardFcn=sigbuilder_block('clipboard');  mask(Sigbuilder block){tuvar=[0:10]}
      mask help: Simulink:masks:SigbuilderBlock_MD
      mask init:
      | if ~strcmp(get_param(bdroot(gcbh),'SimulationStatus'),'stopped') tuvar = sigbuilder_block('maskInit'); end
      settings: CopyFcn=sigbuilder_block('copy');  DeleteFcn=sigbuilder_block('delete');  ModelCloseFcn=sigbuilder_block('modelClose');  PreSaveFcn=sigbuilder_block('preSave');  PauseFcn=sigbuilder_block('pause');  ContinueFcn=sigbuilder_block('continue');  NameChangeFcn=sigbuilder_block('namechange');  OpenFcn=sigbuilder_block('open',[-809.4 12.6 550.8 361.2 ]);  CloseFcn=sigbuilder_block('close');
      mask Display: plot(0, 0, 100, 100,[2, 2, 32, 32, 2], [68, 8, 8, 68, 68],[32, 2], [38, 38], [32, 19, 2],[53, 60, 44], [32, 17, 17, 2],[16, 16, 31, 31]);txt = getActiveGroup(gcbh);text(2, 100, txt,'verticalAlignment', 'top');
  Scope{6,10,12..13} (4 alike) : Scope
  Step5 : Step  Time=GFl_Step_time  Before=GFl_Initial_value  After=GFl_Final_vlaue  SampleTime=GFl_Sample_time
  a : PMIOPort  Side=Right
  b : PMIOPort  Port=2  Side=Right
  c : PMIOPort  Port=3  Side=Right
  wires:
  Bus Selector1/3 -> Gain/1  "<f_PLL>"
  Bus Selector1/2 -> Scope10/1  "<Q_grid>"
  Bus Selector1/1 -> Scope6/1  "<P_grid>"
  Bus Selector1/4 -> Scope13/1  "<V_grid_abc>"
  [conv_1] -> Bus Selector1/1
  Gain/1 -> Scope12/1
  Grid-Following Converter (3-phase)1/1 -> [conv_1]
  Step5/1 -> Grid-Following Converter (3-phase)1/4
  Constant8/1 -> Grid-Following Converter (3-phase)1/1
  P_set_3/1(P_set_1) -> Grid-Following Converter (3-phase)1/2
  Constant9/1 -> Grid-Following Converter (3-phase)1/3
  connections:
  Grid-Following Converter (3-phase)1/RConn3 -- c/RConn1
  Grid-Following Converter (3-phase)1/RConn1 -- a/RConn1
  Grid-Following Converter (3-phase)1/RConn2 -- b/RConn1

== system TEST_simulink/DER 4/Grid Forming Conventer ==
  Bus Selector : BusSelector  OutputSignals=controller.measurements.P_grid,controller.measurements.Q_grid,controller.inner_control.f,physical.V_dc,physical.V_grid_abc
  Constant11 : Constant  Value=GFm_P_primary
  Constant15 : Constant  Value=GFm_Q_set
  Constant16 : Constant  Value=GFmAIC_f_set
  Constant17 : Constant  Value=GFm_V_set_phph
  Grid_Forming_Converter1 : Model_DG_Grid_Forming_Converter/Grid_Forming_Converter  S_n=2e6  V_n_phph=690  f_n=50  send_messages=on  T_s_ctrl=1e-4  T_s_PWM_meas=1e-4  T_s_SPS=1e-4  datatype='double'  swModeling=Average Model  f_sw=5e3  L_filter_conv_pu=[ 0.001 0.05097 ]  C_filter_pu=[ 0.06875 0.04569 ]  L_filter_grid_pu=[ 0.01 0.04 ]  C_dc_pu=0.75  withTransformer=Grid coupling using transformer  V_n_grid_phph=20e3  RL_Trafo_Conv=[ 0.005 0.02 ]  RL_Trafo_Grid=[ 0.005 0.02 ]  Rm=500  Lm=500  meas_lowpass=on  meas_f_cutoff_lowpass=2500  meas_f_cutoff_posseq=20  prot_variant=tDMSquared warnings only  v_dc_max=1.2  v_ac_max=1.4  t_ac_max=0.1  v_ac_maxmax=1.25  t_ac_maxmax=0.1  v_ac_min=0.8  t_ac_min=3  v_ac_minmin=0.45  t_ac_minmin=0.3  f_ac_max=51.5  t_f_ac_max=0.1  f_ac_maxmax=52.5  t_f_ac_maxmax=10  f_ac_min=47.5  t_f_ac_min=0.1  i_ac_max=1.3  outerCtrlStrategy=Droop  OuterCtrl_droop_kP=0.05  OuterCtrl_droop_kQ=0.1  OuterCtrl_droop_TQ=0.2  OuterCtrl_ZDroop_kf=0.05  OuterCtrl_ZDroop_kV=0.1  OuterCtrl_ZDroop_kR=0  OuterCtrl_ZDroop_kX=1  OuterCtrl_ZDroop_TV=0.2  OuterCtrl_VSM_H=0.1  OuterCtrl_VSM_Kd=40  OuterCtrl_VSM_K=20  OuterCtrl_VSM_kQ=0.1  OuterCtrl_VSM_TQ=0.2  OuterCtrl_Dual_Kp=0.01  OuterCtrl_Dual_Kd=1e-4  OuterCtrl_Dual_kQ=0.1  OuterCtrl_Dual_TQ=0.2  OuterCtrl_Lvirt=0  InnerCtrl_K_p_V_cap_controller=0.8  InnerCtrl_K_i_V_cap_controller=0.5  InnerCtrl_K_p_I_conv_controller=3.3  InnerCtrl_K_i_I_conv_controller=16.5  InnerCtrl_v_conv_max=1.3  InnerCtrl_i_conv_max=1  InnerCtrl_Cff_V_cap_ctrl=disabled  InnerCtrl_Cff_I_conv_ctrl=disabled  InnerCtrl_K_ff_I_grid=enabled  InnerCtrl_K_ff_V_cap=enabled  InnerCtrl_i_lim_type=dq coordinate system  InnerCtrl_active_damping=enabled  InnerCtrl_AD_R_virt_pu=0.2
      settings: SourceProductName=tDMSquared
  Ground2 : Ground
  P_set_4 : Subsystem  Tag=STV Subsys  LoadFcn=sigbuilder_block('load');  StartFcn=sigbuilder_block('start');  StopFcn=sigbuilder_block('stop');  ClipboardFcn=sigbuilder_block('clipboard');  mask(Sigbuilder block){tuvar=[0:10]}
      mask help: Simulink:masks:SigbuilderBlock_MD
      mask init:
      | if ~strcmp(get_param(bdroot(gcbh),'SimulationStatus'),'stopped') tuvar = sigbuilder_block('maskInit'); end
      settings: CopyFcn=sigbuilder_block('copy');  DeleteFcn=sigbuilder_block('delete');  ModelCloseFcn=sigbuilder_block('modelClose');  PreSaveFcn=sigbuilder_block('preSave');  PauseFcn=sigbuilder_block('pause');  ContinueFcn=sigbuilder_block('continue');  NameChangeFcn=sigbuilder_block('namechange');  OpenFcn=sigbuilder_block('open',[-809.4 12.6 550.8 361.2 ]);  CloseFcn=sigbuilder_block('close');
      mask Display: plot(0, 0, 100, 100,[2, 2, 32, 32, 2], [68, 8, 8, 68, 68],[32, 2], [38, 38], [32, 19, 2],[53, 60, 44], [32, 17, 17, 2],[16, 16, 31, 31]);txt = getActiveGroup(gcbh);text(2, 100, txt,'verticalAlignment', 'top');
  Scope{1..5} (5 alike) : Scope
  Step4 : Step  Time=GFm_Step_time  Before=GFm_Initial_value  After=GFm_Final_vlaue  SampleTime=GFm_Sample_time
  a : PMIOPort  Side=Right
  b : PMIOPort  Port=2  Side=Right
  c : PMIOPort  Port=3  Side=Right
  wires:
  [conv_1] -> Bus Selector/1
  Grid_Forming_Converter1/1 -> [conv_1]
  Bus Selector/4 -> Scope4/1  "<V_dc>"
  Bus Selector/1 -> Scope1/1  "<P_grid>"
  Bus Selector/3 -> Scope3/1  "<f>"
  Bus Selector/2 -> Scope2/1  "<Q_grid>"
  Bus Selector/5 -> Scope5/1  "<V_grid_abc>"
  Constant15/1 -> Grid_Forming_Converter1/3
  Ground2/1 -> Grid_Forming_Converter1/6
  Step4/1 -> Grid_Forming_Converter1/7
  Constant17/1 -> Grid_Forming_Converter1/5
  P_set_4/1(P_set_1) -> Grid_Forming_Converter1/2
  Constant11/1 -> Grid_Forming_Converter1/1
  Constant16/1 -> Grid_Forming_Converter1/4
  connections:
  Grid_Forming_Converter1/RConn3 -- c/RConn1
  Grid_Forming_Converter1/RConn1 -- a/RConn1
  Grid_Forming_Converter1/RConn2 -- b/RConn1

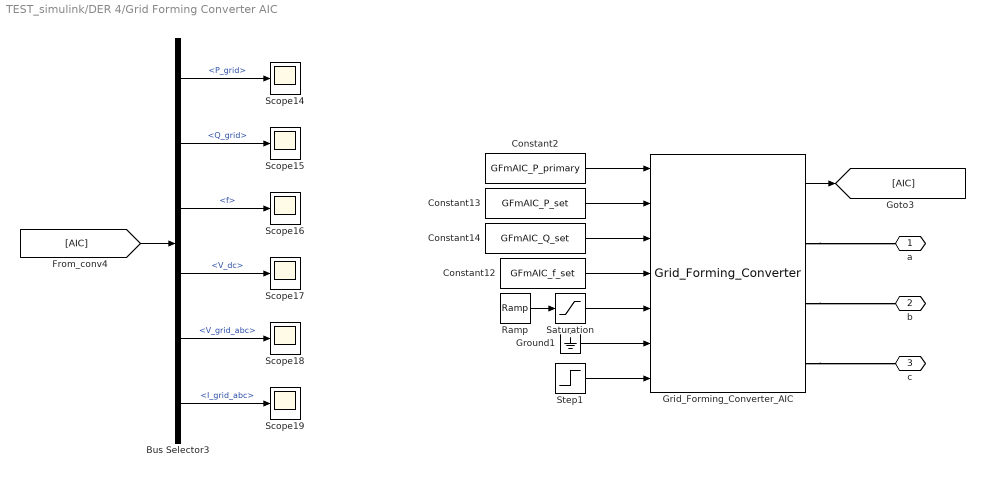
== system TEST_simulink/DER 4/Grid Forming Converter AIC ==
  Bus Selector3 : BusSelector  OutputSignals=controller.measurements.P_grid,controller.measurements.Q_grid,controller.inner_control.f,physical.V_dc,physical.V_grid_abc,physical.I_grid_abc
  Constant12 : Constant  Value=GFmAIC_f_set
  Constant13 : Constant  Value=GFmAIC_P_set
  Constant14 : Constant  Value=GFmAIC_Q_set
  Constant2 : Constant  Value=GFmAIC_P_primary
  Grid_Forming_Converter_AIC : Model_DG_Grid_Forming_Converter/Grid_Forming_Converter  S_n=100e3  V_n_phph=400  f_n=50  send_messages=on  T_s_ctrl=2e-4  T_s_PWM_meas=1e-5  T_s_SPS=1e-5  datatype='double'  swModeling=Average Model  f_sw=2.5e3  L_filter_conv_pu=[ 0.001 0.0177 ]  C_filter_pu=[ 0.000104 0.213 ]  L_filter_grid_pu=[ 0.001 0.00432 ]  C_dc_pu=0.75  withTransformer=Direct grid coupling of converter  V_n_grid_phph=400  RL_Trafo_Conv=[ 0.005 0.02 ]  RL_Trafo_Grid=[ 0.005 0.02 ]  Rm=500  Lm=500  meas_lowpass=on  meas_f_cutoff_lowpass=2500  meas_f_cutoff_posseq=20  prot_variant=tDMSquared warnings only  v_dc_max=1.2  v_ac_max=1.4  t_ac_max=0.1  v_ac_maxmax=1.25  t_ac_maxmax=0.1  v_ac_min=0.8  t_ac_min=3  v_ac_minmin=0.45  t_ac_minmin=0.3  f_ac_max=51.5  t_f_ac_max=0.1  f_ac_maxmax=52.5  t_f_ac_maxmax=10  f_ac_min=47.5  t_f_ac_min=0.1  i_ac_max=1.3  outerCtrlStrategy=Droop  OuterCtrl_droop_kP=0.05  OuterCtrl_droop_kQ=0.1  OuterCtrl_droop_TQ=0.2  OuterCtrl_ZDroop_kf=0.05  OuterCtrl_ZDroop_kV=0.1  OuterCtrl_ZDroop_kR=0  OuterCtrl_ZDroop_kX=1  OuterCtrl_ZDroop_TV=0.2  OuterCtrl_VSM_H=0.1  OuterCtrl_VSM_Kd=40  OuterCtrl_VSM_K=20  OuterCtrl_VSM_kQ=0.1  OuterCtrl_VSM_TQ=0.2  OuterCtrl_Dual_Kp=0.01  OuterCtrl_Dual_Kd=1e-4  OuterCtrl_Dual_kQ=0.1  OuterCtrl_Dual_TQ=0.2  OuterCtrl_Lvirt=0  InnerCtrl_K_p_V_cap_controller=0.17  InnerCtrl_K_i_V_cap_controller=4.24  InnerCtrl_K_p_I_conv_controller=0.5  InnerCtrl_K_i_I_conv_controller=2.5  InnerCtrl_v_conv_max=1.3  InnerCtrl_i_conv_max=1.32  InnerCtrl_Cff_V_cap_ctrl=disabled  InnerCtrl_Cff_I_conv_ctrl=disabled  InnerCtrl_K_ff_I_grid=enabled  InnerCtrl_K_ff_V_cap=enabled  InnerCtrl_i_lim_type=abc coordinate system  InnerCtrl_active_damping=enabled  InnerCtrl_AD_R_virt_pu=0.1
      settings: SourceProductName=tDMSquared
  Ground1 : Ground
  Ramp : simulink/Sources/Ramp  slope=400  start=0  InitialOutput=0
  Saturation : Saturate  UpperLimit=400
  Scope{14..19} (6 alike) : Scope
  Step1 : Step  Time=GFmAIC_Step_time  Before=GFmAIC_Initial_value  After=GFmAIC_Final_vlaue  SampleTime=GFmAIC_Sample_time
  a : PMIOPort  Side=Right
  b : PMIOPort  Port=2  Side=Right
  c : PMIOPort  Port=3  Side=Right
  wires:
  Bus Selector3/1 -> Scope14/1  "<P_grid>"
  Bus Selector3/4 -> Scope17/1  "<V_dc>"
  Bus Selector3/3 -> Scope16/1  "<f>"
  Grid_Forming_Converter_AIC/1 -> [AIC]
  Bus Selector3/5 -> Scope18/1  "<V_grid_abc>"
  [AIC] -> Bus Selector3/1
  Bus Selector3/6 -> Scope19/1  "<I_grid_abc>"
  Bus Selector3/2 -> Scope15/1  "<Q_grid>"
  Constant13/1 -> Grid_Forming_Converter_AIC/2
  Saturation/1 -> Grid_Forming_Converter_AIC/5
  Constant2/1 -> Grid_Forming_Converter_AIC/1
  Ramp/1 -> Saturation/1
  Constant12/1 -> Grid_Forming_Converter_AIC/4
  Ground1/1 -> Grid_Forming_Converter_AIC/6
  Constant14/1 -> Grid_Forming_Converter_AIC/3
  Step1/1 -> Grid_Forming_Converter_AIC/7
  connections:
  Grid_Forming_Converter_AIC/RConn3 -- c/RConn1
  Grid_Forming_Converter_AIC/RConn1 -- a/RConn1
  Grid_Forming_Converter_AIC/RConn2 -- b/RConn1

== system TEST_simulink/DER 4/SG ==
  Bus Selector2 : BusSelector  OutputSignals=electrical_SI.P_grid_SI,electrical_SI.Q_grid_SI,SG_SI.Frequency (Hz),electrical_SI.V_grid_SI
  Constant1 : Constant  Value=SG_P_primary
  Constant3 : Constant  Value=SG_f_set
  Constant5 : Constant  Value=SG_Q_set
  Constant7 : Constant  Value=SG_V_set_phph
  P_set_2 : Subsystem  Tag=STV Subsys  LoadFcn=sigbuilder_block('load');  StartFcn=sigbuilder_block('start');  StopFcn=sigbuilder_block('stop');  ClipboardFcn=sigbuilder_block('clipboard');  mask(Sigbuilder block){tuvar=[0:10]}
      mask help: Simulink:masks:SigbuilderBlock_MD
      mask init:
      | if ~strcmp(get_param(bdroot(gcbh),'SimulationStatus'),'stopped') tuvar = sigbuilder_block('maskInit'); end
      settings: CopyFcn=sigbuilder_block('copy');  DeleteFcn=sigbuilder_block('delete');  ModelCloseFcn=sigbuilder_block('modelClose');  PreSaveFcn=sigbuilder_block('preSave');  PauseFcn=sigbuilder_block('pause');  ContinueFcn=sigbuilder_block('continue');  NameChangeFcn=sigbuilder_block('namechange');  OpenFcn=sigbuilder_block('open',[665.4 126 550.8 400.2 ]);  CloseFcn=sigbuilder_block('close');
      mask Display: plot(0, 0, 100, 100,[2, 2, 32, 32, 2], [68, 8, 8, 68, 68],[32, 2], [38, 38], [32, 19, 2],[53, 60, 44], [32, 17, 17, 2],[16, 16, 31, 31]);txt = getActiveGroup(gcbh);text(2, 100, txt,'verticalAlignment', 'top');
  Scope{7..9,11} (4 alike) : Scope
  Step2 : Step  Time=SG_Step_time  Before=SG_Initial_value  After=SG_Final_vlaue  SampleTime=SG_Sample_time
  Synchronous_Generator : Model_DG_Synchronous_Generator/Synchronous_Generator  S_n=3.2e6  P_binst=2.0e6  V_n_phph=400  V_n_grid_phph=20e3  f_n=50  T_s_ctrl=1e-4  T_s_meas=1e-4  datatype='double'  SG_Reactances=[ 3.19 0.33 0.159 1.79 0.155 0.05 ]  SG_TimeConstants=[ 0.5 0.025 0.025 ]  SG_StatorResistance=0.00074  SG_mech=[ 0.366 0.01 2 ]  gov_type=IEEEG1 simplified  K_IEEEG1simp=10  T_IEEEG1simp=[ 0.2 0 0.1 0 ]  dP_maxmin_IEEEG1simp=[ 2 -2 ]  exciterModel=AC1A  QCtrl=Constant Voltage (no Q-Control)  K_p_QCtrl=0.5  K_i_QCtrl=0.4  uq0ref=1.0  qmax=0.33  umax=1.04  deadband=0  p_pu=[0.1, 0.5, 0.6, 0.9, 1.0]  q_pu=[0.0, 0.0, -0.05, -0.33, -0.33]  p1=[0.94, 0.33]  p2=[0.96, 0]  p3=[1.04, 0]  p4=[1.06, -0.33]  cosphi_ref=1  ind_cap_Q=Inductive behavior (capacitive Q infeed)  use_transformer=Grid coupling with transformer  RL_Trafo_GenSide=[ 0.002 0.08 ]  RL_Trafo_GridSide=[ 0.002 0.08 ]  Trafo_RmLm=[ 500 500 ]
      link override SG_Control/Exciter: LabelModeActiveChoice=AC1A
      link override SG_Control/Reactive_Power_Controller: LabelModeActiveChoice=const_V
      settings: SourceProductName=tDMSquared
  a : PMIOPort  Side=Right
  b : PMIOPort  Port=2  Side=Right
  c : PMIOPort  Port=3  Side=Right
  wires:
  Synchronous_Generator/1 -> [sg]
  [sg] -> Bus Selector2/1
  Bus Selector2/3 -> Scope9/1  "<Frequency (Hz)>"
  Bus Selector2/1 -> Scope7/1  "<P_grid_SI>"
  Bus Selector2/2 -> Scope8/1  "<Q_grid_SI>"
  Bus Selector2/4 -> Scope11/1  "<V_grid_SI>"
  Constant7/1 -> Synchronous_Generator/5
  Constant3/1 -> Synchronous_Generator/4
  Constant1/1 -> Synchronous_Generator/1
  P_set_2/1(P_set_2) -> Synchronous_Generator/2
  Step2/1 -> Synchronous_Generator/6
  Constant5/1 -> Synchronous_Generator/3
  connections:
  Synchronous_Generator/RConn3 -- c/RConn1
  Synchronous_Generator/RConn1 -- a/RConn1
  Synchronous_Generator/RConn2 -- b/RConn1

== system TEST_simulink/DER 5/Grid Following Conventer ==
  Bus Selector1 : BusSelector  OutputSignals=controller.measurements.P_grid,controller.measurements.Q_grid,controller.PLL.f_PLL,physical.V_grid_abc
  Constant8 : Constant  Value=GFl_P_primary
  Constant9 : Constant  Value=GFl_Q_set
  Gain : Gain  Gain=50
  Grid-Following Converter (3-phase)1 : Model_DG_Grid_Following_Converter/Grid-Following Converter (3-phase)  S_n=2e6  P_binst=1.5e6  V_n_phph=690  f_n=50  send_messages=on  T_s_ctrl=1e-3  T_s_PWM_meas=1e-4  T_s_SPS=1e-4  datatype='double'  swModeling=Average Model  f_sw=5e3  L_filter_conv_pu=[ 0.005 0.23 ]  C_filter_pu=[ 0.005 0.01 ]  L_filter_grid_pu=[ 0.01 0.04 ]  withTransformer=Grid coupling using transformer  V_n_grid_phph=20e3  RL_Trafo_Conv=[ 0.005 0.02 ]  RL_Trafo_Grid=[ 0.005 0.02 ]  Rm=500  Lm=500  meas_LPF=on  meas_LPF_f_cutoff=2500  prot_variant=tDMSquared warnings only  prot_v_ac_max=1.4  prot_t_ac_max=0.1  prot_v_ac_maxmax=1.25  prot_t_ac_maxmax=0.1  prot_v_ac_min=0.8  prot_t_ac_min=3  prot_v_ac_minmin=0.45  prot_t_ac_minmin=0.3  prot_f_ac_max=51.5  prot_t_f_ac_max=0.1  prot_f_ac_maxmax=52.5  prot_t_f_ac_maxmax=10  prot_f_ac_min=47.5  prot_t_f_ac_min=0.1  prot_i_ac_max=1.3  unitCtrlMode=VDE 4110  VDE4110_Pf_DBlow=49.8  VDE4110_Pf_DBhigh=50.2  VDE4110_Pf_droop=5  VDE4110_Pf_dPdt_max=1  VDE4110_Pf_T_LPF=33e-3  VDE4110_Pf_isStorage=on  VDE4110_Q_Mode=(c) Constant Q with Q(V)-limitation  VDE4110_Q_T_PT1=3.33  VDE4110_uq0ref=1  VDE4110_qmax=0.33  VDE4110_umax=1.04  VDE4110_deadband=0  VDE4110_p_pu=[0.1, 0.5, 0.6, 0.9, 1.0]  VDE4110_q_pu=[0.0, 0.0, -0.05, -0.33, -0.33]  VDE4110_p1=[0.94, 0.33]  VDE4110_p2=[0.96, 0]  VDE4110_p3=[1.04, 0]  VDE4110_p4=[1.06, -0.33]  VDE4110_cosphi_ref=1  VDE4110_Q_direction=Inductive Q injection  InnerCtrl_PQ_Ctrl_Mode=Closed loop  InnerCtrl_Kp_PQ=1  InnerCtrl_Ki_PQ=5  InnerCtrl_Kp=0.3  InnerCtrl_Ki=2  InnerCtrl_v_conv_max=1.25  InnerCtrl_i_conv_max=1.1  InnerCtrl_AD_activated=on  InnerCtrl_AD_Rvirt=0.1
      settings: SourceProductName=tDMSquared
  P_set_3 : Subsystem  Tag=STV Subsys  LoadFcn=sigbuilder_block('load');  StartFcn=sigbuilder_block('start');  StopFcn=sigbuilder_block('stop');  ClipboardFcn=sigbuilder_block('clipboard');  mask(Sigbuilder block){tuvar=[0:10]}
      mask help: Simulink:masks:SigbuilderBlock_MD
      mask init:
      | if ~strcmp(get_param(bdroot(gcbh),'SimulationStatus'),'stopped') tuvar = sigbuilder_block('maskInit'); end
      settings: CopyFcn=sigbuilder_block('copy');  DeleteFcn=sigbuilder_block('delete');  ModelCloseFcn=sigbuilder_block('modelClose');  PreSaveFcn=sigbuilder_block('preSave');  PauseFcn=sigbuilder_block('pause');  ContinueFcn=sigbuilder_block('continue');  NameChangeFcn=sigbuilder_block('namechange');  OpenFcn=sigbuilder_block('open',[-809.4 12.6 550.8 361.2 ]);  CloseFcn=sigbuilder_block('close');
      mask Display: plot(0, 0, 100, 100,[2, 2, 32, 32, 2], [68, 8, 8, 68, 68],[32, 2], [38, 38], [32, 19, 2],[53, 60, 44], [32, 17, 17, 2],[16, 16, 31, 31]);txt = getActiveGroup(gcbh);text(2, 100, txt,'verticalAlignment', 'top');
  Scope{6,10,12..13} (4 alike) : Scope
  Step5 : Step  Time=GFl_Step_time  Before=GFl_Initial_value  After=GFl_Final_vlaue  SampleTime=GFl_Sample_time
  a : PMIOPort  Side=Right
  b : PMIOPort  Port=2  Side=Right
  c : PMIOPort  Port=3  Side=Right
  wires:
  Bus Selector1/3 -> Gain/1  "<f_PLL>"
  Bus Selector1/2 -> Scope10/1  "<Q_grid>"
  Bus Selector1/1 -> Scope6/1  "<P_grid>"
  Bus Selector1/4 -> Scope13/1  "<V_grid_abc>"
  [conv_1] -> Bus Selector1/1
  Gain/1 -> Scope12/1
  Grid-Following Converter (3-phase)1/1 -> [conv_1]
  Step5/1 -> Grid-Following Converter (3-phase)1/4
  Constant8/1 -> Grid-Following Converter (3-phase)1/1
  P_set_3/1(P_set_1) -> Grid-Following Converter (3-phase)1/2
  Constant9/1 -> Grid-Following Converter (3-phase)1/3
  connections:
  Grid-Following Converter (3-phase)1/RConn3 -- c/RConn1
  Grid-Following Converter (3-phase)1/RConn1 -- a/RConn1
  Grid-Following Converter (3-phase)1/RConn2 -- b/RConn1
